simulink model "hcu_main_ADASwEPS"  (Simulink 8.2)
settings: Solver=FixedStepDiscrete  StartTime=0.0  StopTime=inf  FixedStep=0.001  RelTol=1e-3
PostLoadFcn:
  | , if any(exist('dsrtsu_mdlpostloadfcn', 'file') == [2, 3, 6]), try dsrtsu_mdlpostloadfcn('Execute', bdroot); catch fprintf('Error in PostLoadFcn (dsrtsu_mdlpostloadfcn) for model "%s":\n %s\n', bdroot, lasterr); end, end,
values from neighbouring files (symbols this model uses):
  C_TASK_1MS_S = (	C_TICK_TIME_S       )    [hcu_local_hdr.m]    (also in temp_ovrd_values.m = double(	0.001                  ))
  C_TASK_5MS_S = (	C_TICK_TIME_S      	)    [hcu_local_hdr.m]
  ENUM_ADASLFCSTATUS_OFF = uint8(  0  )    [hcu_local_hdr.m]
  ENUM_ADASLFCSTATUS_STANDBY = uint8(  1  )    [hcu_local_hdr.m]
  ENUM_ADASLKASTATUS_ACTIVE = uint8(  2  )    [hcu_local_hdr.m]
  ENUM_ADASLKASTATUS_OFF = uint8(  0  )    [hcu_local_hdr.m]
  ENUM_ADASLKASTATUS_STANDBY = uint8(  1  )    [hcu_local_hdr.m]
  ENUM_EPSMODEREQ_ANGLE = uint8(  1  )    [hcu_local_hdr.m]
  ENUM_EPSMODEREQ_INTERNAL = uint8(  0  )    [hcu_local_hdr.m]
  ENUM_EPSMODEREQ_TORQUE = uint8(  2  )    [hcu_local_hdr.m]
  ENUM_GEARPOSN_1ST = uint8(  1  )    [hcu_local_hdr.m]
  ENUM_GEARPOSN_2ND = uint8(  2  )    [hcu_local_hdr.m]
  ENUM_GEARPOSN_3RD = uint8(  3  )    [hcu_local_hdr.m]
  ENUM_GEARPOSN_4TH = uint8(  4  )    [hcu_local_hdr.m]
  ENUM_GEARPOSN_5TH = uint8(  5  )    [hcu_local_hdr.m]
  ENUM_GEARPOSN_6TH = uint8(  6  )    [hcu_local_hdr.m]
  ENUM_GEARPOSN_PN = uint8(  0  )    [hcu_local_hdr.m]
  ENUM_GEARPOSN_R = uint8(  7  )    [hcu_local_hdr.m]
  FALSE = boolean( 0 )    [hcu_local_hdr.m]
  TRUE = boolean( 1 )    [hcu_local_hdr.m]
undefined symbols (not defined in the file or in its folder): AACC_DistCtrlIMult_X_mps2, AACC_DistCtrlPMult_X_mps2, AACC_GearActual_enum, AACC_SpdCtrlIMult_X_mps2, AACC_SpdCtrlPMult_X_mps2, AACC_VehSpd_kph, AISP_EPSCurrent_pct, AISP_TqASensorDelta_pct, AISP_TqBSensorDelta_pct, ENUM_ACCSTATUS_ACTIVE, ENUM_ACCSTATUS_OFF, ENUM_ACCSTATUS_STANDBY, ENUM_ADASLFCSTATUS_ACTIVE, ENUM_ADASLFCSTATUS_TRANSITION, ENUM_LFCCCONTSTATUS_ACTIVE, ENUM_LFCCCONTSTATUS_NOTAVAIL_TEMP, ENUM_LFCCCONTSTATUS_OFF, ENUM_LFCCCONTSTATUS_READY, ENUM_LFCCCONTSTATUS_TRANSITION, ENUM_LKACCONTSTATUS_ACTIVE, ENUM_LKACCONTSTATUS_NOTAVAIL_TEMP, ENUM_LKACCONTSTATUS_OFF, ENUM_LKACCONTSTATUS_READY, KACC_AcclReqMax_g, KACC_AcclReqMin_g, KACC_ACCSetTimeGapDef1_s, KACC_ACCSetTimeGapDef2_s, KACC_ACCSetTimeGapDef3_s, KACC_ACCSetTimeGapDef4_s, KACC_ACCSetTimeGapDef5_s, KACC_AirDensity_kgpm3, KACC_AirDragCoef_rat, KACC_CommandsOn_flg, KACC_CruzSpdChgTimeThres_s, KACC_DecReqSwOffThres_Nm, KACC_DecReqSwOnThres_Nm, KACC_DistCtrlAdjTime_s, KACC_DistCtrlCalRate_s, KACC_DistCtrlIC_mps2, KACC_DistCtrlIGain_rat, KACC_DistCtrlIMax_mps2, KACC_DistCtrlIMin_mps2, KACC_DistCtrlIRest_flg, KACC_DistCtrlKGain_rat, KACC_DistCtrlPause_flg, KACC_DistCtrlPGain_rat, KACC_FinalDriveEff_pct, KACC_FinalDriveRatio_rat, KACC_FrontalArea_m2, KACC_GearBoxEff_pct, KACC_LongPushSpdChg_kph, KACC_MaxAccSetSpd_kph, KACC_MinAccSetSpd_kph, KACC_SetAllowSpdLim_kph, KACC_SpdCtrlAdjTime_s, KACC_SpdCtrlCalRate_s, KACC_SpdCtrlIC_mps2, KACC_SpdCtrlIGain_rat, KACC_SpdCtrlIMax_mps2, KACC_SpdCtrlIMin_mps2 ... (+26)
libraries: simulink x54, adas_lib x6, rti1401lib_dio_type3 x4, rtimmsu_dsrtlib x3, hcu_lib x2, aeb x1, ddm x1, dfr x1, dgi x1, dhp x1, dinr x1, dip x1
(part 1 of 9)
settings Model: DSRTSU_INTERNAL_RTI_VER=460  DSRTSU_INTERNAL_RTI_TYPE=rti1401  RTICANMMDATA=struct('GeneralSetupData',struct('modelroot','D:\HAITEC\SVN\trunk\ADAS_Softwares\HTDragon\software\sw_development\arch','generalsettings',struct('filesettings',struct('destfolder',struct('Name','..\build\RTICANMM_FILES_ADASwEPS','Check',1),'buildfolder',struct('Name','.','Check',1),'AbsDestfolder',struct('Name','D:\HAITEC\SVN\trunk\ADAS_Softwares\HTDragon\software\sw_development\build\RTICANMM_FILES_ADASwEPS'),'AbsBuildfolder',struct('Name','D:\HAITEC\SVN\trunk\ADAS_Softwares\HTDragon\software\sw_development\arch'))),'options',struct('addpaths',1,'rmpaths',1,'addtrcexclusion',1,'cannavigator',struct('checkmonitoring',1),'show_usrtrc',0,'use_usrtrc',0,'addpath2usrmk',1),'advanced',struct('options',[1 1 1 1 1 1 1 1 1 1 1 1 1 1 1 1 1 1 1 1 1 1 1 1 1 1 1 1 1 1 1 1 1 1 1 1 1 1 1 1 1 1 1 1 1 1 1 1 1 1 1 1 1 1 1 1 1 1 1 1 1 1 1 1 1 1 1 1 1 1 1 1 1 1 1 1 1 1 1 1 1 1 1 1 1 1 1 1 1 1 1 1 1 1 1 1 1 1 1 1]),'MPSetup',{{}},'modelname','hcu_main_ADASwEPS','blockdata',struct('generalsettings',struct('filesettings',struct('destfolder',struct('Name','.','Check',1),'AbsDestfolder',struct('Name','T:\TOOL_SOURCES\CANnedy\m'),'buildfolder',struct('Name','.','Check',1),'AbsBuildfolder',struct('Name','C:\MATLAB6p5\work'))),'options',struct('addpaths',1,'rmpaths',1,'addpath2usrmk',1),'modelname','rticanmmlib','modelroot','T:\TOOL_SOURCES\CANnedy\m'),'MMType','RTICANMM','block',['hcu_main_ADASwEPS/RTICANMM' char(10) 'GeneralSetup'],'userdata',struct('HostServiceChannelID',{{'CAN_2',[],'CAN_1'}}),'RTI',struct('Type','RTI1401','Ver','7.4','Date','02-May-2015'),'version','4.1.736021.4900694444'))  DSRTSU_INTERNAL_RTIFPGA=50  Creator=11116  LastModifiedBy=14014  BufferReuse=off
settings DataIOCC: SignalLoggingSaveFormat=Dataset  SaveOutput=off  SaveTime=off
settings OptimizationCC: BlockReduction=off  OptimizeBlockIOStorage=off  BufferReuse=off  ExpressionFolding=off  ExpressionDepthLimit=128  LocalBlockOutputs=off
settings DebuggingCC: ParameterPrecisionLossMsg=none  FcnCallInpInsideContextMsg=EnableAllAsError  StateNameClashWarn=none
settings HardwareCC: ProdIntDivRoundTo=Zero  ProdEndianess=BigEndian  ProdHWDeviceType=Generic->Custom  TargetIntDivRoundTo=Zero  TargetEndianess=BigEndian  TargetHWDeviceType=Generic->Custom
settings RTWCC: SystemTargetFile=rti1401.tlc  MakeCommand=make_rti  TemplateMakefile=rti1401.tmf  Description=dSPACE DS1401 Hardware Platform  ProcessScript=rti1401_make_rtw_hook
settings STFCustomTargetCC: CodeReplacementLibrary=ANSI_C  ParMdlRefBuildCompliant=on  GeneratePreprocessorConditionals=Disable all  SystemTargetFile=rti1401.tlc
settings GRTTargetCC: CompOptLevelCompliant=off  ConcurrentExecutionCompliant=off  MatFileLogging=off  ExtModeMexFile=noextcomm
settings CustomProperty: DataType=RTWOptions_EnumType_C__Program Files_dSPACE RCPHIL 2015-A_MATLAB_RTI_RTI1401_TLC_rti1401_1InitialSimState  Value=RUN
settings EnumStrPairs: String=RUN

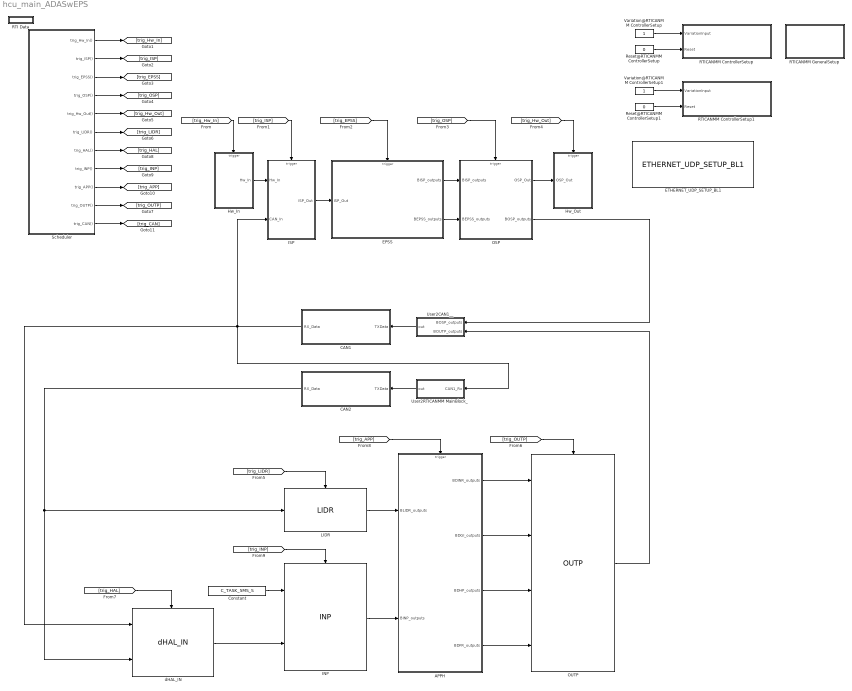
== system hcu_main_ADASwEPS ==
  APPH : Subsystem
      settings: RTWSystemCode=Nonreusable function  RTWFcnNameOpts=Use subsystem name  RTWFileNameOpts=Use subsystem name
  CAN1 : Subsystem  InitFcn=rticanmm_blockfcn('InitFcn', 'CANnedy', gcb)  ClipboardFcn=rticanmm_blockfcn('ClipboardFcn', 'CANnedy', gcb)  mask(RTICANMM){DSProperties=struct('RTI',struct('Version',uint32(1),'BlockType',struct('isSLSource',uint8(1),'isSLSink',uint8(1),'isHWSource',uint8(0),'isHWSink',uint8(0),'isSetup',uint8(0),'isInline',uint8(1),'isNonInline',uint8(0),'isInterrupt',uint8(0),'isChannelwise',uint8(0)),'IOBoardType','RTICANMM','UnitType','RTICANMM','Identifier','Mainblock','DialogType','SL','BlockSet','RTICANMM','SlaveProcessor','CAN')), CANMMProperties=struct('RTICANMMVersion','4.1','RTICANMMVersionIntern','4.1.736021.4900694444','RTICANMMDate','02-May-2015','Settings','RTICANMM_MAIN_CAN_1','UserTracePath','','ModelPath','D:\HAITEC\SVN\trunk\ADAS_Softwares\HTDragon\software\sw_development\arch','filesettings',struct('FileName','..\..\..\..\CAN\ADAS_CAN1_Mule1_BSGEMS_MVCU_MEPS_20160121_db.dbc','IsRelative',1,'ClusterId',1,'ClusterList',{{'default'}},'destfolder',struct('Name','..\build\RTICANMM_FILES_ADASwEPS','Check',1),'buildfolder',struct('Name','.','Check',1),'onlyfreerawcapture',0,'overlapping2variant',0,'canfdsupport',0,'shortestJ2container',1),'onlyfreerawcapture',0,'Board',['CAN Type 1'],'BoardNum','1','ChannelNum','1','Variation','1','SetupId','CAN_1','MARK',['87FB4930AEF4A7AAC589F26C78E4F4';'72FEF8353FB46D1087126C7939F170';'8EAD2A2CD2FE1AE61023D4FA11BE9C';'5611A927C2EC9CAF50988DCF8D639B';'13F55C241594A2B2B8AC667E2018BB'],'date','23-Jan-2016','clock',['23.01.2016 09:32:58'],'recreate',0,'RTIVER','RTI1401','j1939',0,'TRC',struct('include',1),'rtsupport',struct('XMLFile','D:\HAITEC\SVN\trunk\ADAS_Softwares\HTDragon\software\sw_development\build\RTICANMM_FILES_ADASwEPS\RTICANMM_MAIN_CAN_1.xml','DBCXML',struct('Path','D:\HAITEC\SVN\trunk\ADAS_Softwares\HTDragon\software\sw_development\build\RTICANMM_FILES_ADASwEPS\RTICANMM_MAIN_CAN_1_dbc.xml','support',1,'Name','ADAS_CAN1_Mule1_BSGEMS_MVCU_MEPS_20160121_db.dbc','Date',['22-一月-2016 09:11:58'],'Type','standard','DBCSupport','ON'))), CANMMType=CANnedy, CANMMUserTraceMerged=off, CANMMUserTracePath=, CANMMChannelNum=1, CANMMBoardNum=1, CANMMDestFolder=..\build\RTICANMM_FILES_ADASwEPS, CANMMFolder=., CANMMSetupId=CAN_1, CANMMsave2mat=['87FB4930AEF4A7AAC589F26C78E4F4';'72FEF8353FB46D1087126C7939F170';'8EAD2A2CD2FE1AE61023D4FA11BE9C';'5611A927C2EC9CAF50988DCF8D639B';'13F55C241594A2B2B8AC667E2018BB'], CANMMName=CAN_1, CANMMSettings=RTICANMM_MAIN_CAN_1, CANMMIntermediateTag=RTICANMM_MAIN_CAN_1_intermediate, CANMMsfcnname=RTICANMM_MAIN_CAN_1}
      mask init:
      | rticanmm_initfcn(gcb, CANMMType, CANMMsfcnname)
      settings: AttributesFormatString=CAN_1[CAN_1]: DS1401_B1_C1_V1  CopyFcn=rticanmm_blockfcn('CopyFcn', 'CANnedy', gcb)  DeleteFcn=rticanmm_blockfcn('DeleteFcn', 'CANnedy', gcb)  ModelCloseFcn=rticanmm_blockfcn('ModelCloseFcn', 'CANnedy', gcb)  NameChangeFcn=rticanmm_blockfcn('NameChangeFcn', 'CANnedy', gcb)  OpenFcn=try, rticanmm_main_gui('create',gcb); ; catch,errordlg({lasterr, '','Please check your RTI installation.'},['Error: ' upper(bdroot)], 'replace'); end  MoveFcn=rticanmm_blockfcn('MoveFcn', 'CANnedy', gcb)
      mask Help: eval('rticanmm_quickstart(''create'', gcb);', 'disp(lasterr);')
      mask Display:
      | disp(sprintf('RTI CAN\nMultiMessage\nMainSetup'))
      | port_label('input', 1, 'TX Data')
      | port_label('output', 1, 'RX Data')
  CAN2 : Subsystem  InitFcn=rticanmm_blockfcn('InitFcn', 'CANnedy', gcb)  ClipboardFcn=rticanmm_blockfcn('ClipboardFcn', 'CANnedy', gcb)  mask(RTICANMM){DSProperties=struct('RTI',struct('Version',uint32(1),'BlockType',struct('isSLSource',uint8(1),'isSLSink',uint8(1),'isHWSource',uint8(0),'isHWSink',uint8(0),'isSetup',uint8(0),'isInline',uint8(1),'isNonInline',uint8(0),'isInterrupt',uint8(0),'isChannelwise',uint8(0)),'IOBoardType','RTICANMM','UnitType','RTICANMM','Identifier','Mainblock','DialogType','SL','BlockSet','RTICANMM','SlaveProcessor','CAN')), CANMMProperties=struct('RTICANMMVersion','4.1','RTICANMMVersionIntern','4.1.736021.4900694444','RTICANMMDate','02-May-2015','Settings','RTICANMM_MAIN_CAN_2','UserTracePath','','ModelPath','D:\HAITEC\SVN\trunk\ADAS_Softwares\HTDragon\software\sw_development\arch','filesettings',struct('FileName','..\..\..\..\CAN\IDIADA_CAN2_Chimo.dbc','IsRelative',1,'ClusterId',1,'ClusterList',{{'default'}},'destfolder',struct('Name','..\build\RTICANMM_FILES_ADASwEPS','Check',1),'buildfolder',struct('Name','.','Check',1),'onlyfreerawcapture',0,'overlapping2variant',0,'canfdsupport',0,'shortestJ2container',1),'onlyfreerawcapture',0,'Board',['CAN Type 1'],'BoardNum','1','ChannelNum','2','Variation','1','SetupId','CAN_2','MARK',['4E53C812CB570F3DF79E35A61EC1B4';'A1237348498B5F46CB73D5EF117ED2';'77465375665041D5559DC8396B874D';'03CE9519A3063C2C69A49AF64F1FBA';'05E25404A442834EF54FA0177E6CB6'],'date','23-Jan-2016','clock',['23.01.2016 09:38:04'],'recreate',0,'RTIVER','RTI1401','j1939',0,'TRC',struct('include',1),'rtsupport',struct('XMLFile','D:\HAITEC\SVN\trunk\ADAS_Softwares\HTDragon\software\sw_development\build\RTICANMM_FILES_ADASwEPS\RTICANMM_MAIN_CAN_2.xml','DBCXML',struct('Path','D:\HAITEC\SVN\trunk\ADAS_Softwares\HTDragon\software\sw_development\build\RTICANMM_FILES_ADASwEPS\RTICANMM_MAIN_CAN_2_dbc.xml','support',1,'Name','IDIADA_CAN2_Chimo.dbc','Date',['23-一月-2016 09:07:49'],'Type','standard','DBCSupport','ON'))), CANMMType=CANnedy, CANMMUserTraceMerged=off, CANMMUserTracePath=, CANMMChannelNum=2, CANMMBoardNum=1, CANMMDestFolder=..\build\RTICANMM_FILES_ADASwEPS, CANMMFolder=., CANMMSetupId=CAN_2, CANMMsave2mat=['4E53C812CB570F3DF79E35A61EC1B4';'A1237348498B5F46CB73D5EF117ED2';'77465375665041D5559DC8396B874D';'03CE9519A3063C2C69A49AF64F1FBA';'05E25404A442834EF54FA0177E6CB6'], CANMMName=CAN_2, CANMMSettings=RTICANMM_MAIN_CAN_2, CANMMIntermediateTag=RTICANMM_MAIN_CAN_2_intermediate, CANMMsfcnname=RTICANMM_MAIN_CAN_2}
      mask init:
      | rticanmm_initfcn(gcb, CANMMType, CANMMsfcnname)
      settings: AttributesFormatString=CAN_2[CAN_2]: DS1401_B1_C2_V1  CopyFcn=rticanmm_blockfcn('CopyFcn', 'CANnedy', gcb)  DeleteFcn=rticanmm_blockfcn('DeleteFcn', 'CANnedy', gcb)  ModelCloseFcn=rticanmm_blockfcn('ModelCloseFcn', 'CANnedy', gcb)  NameChangeFcn=rticanmm_blockfcn('NameChangeFcn', 'CANnedy', gcb)  OpenFcn=try, rticanmm_main_gui('create',gcb); ; catch,errordlg({lasterr, '','Please check your RTI installation.'},['Error: ' upper(bdroot)], 'replace'); end  MoveFcn=rticanmm_blockfcn('MoveFcn', 'CANnedy', gcb)
      mask Help: eval('rticanmm_quickstart(''create'', gcb);', 'disp(lasterr);')
      mask Display:
      | disp(sprintf('RTI CAN\nMultiMessage\nMainSetup'))
      | port_label('input', 1, 'TX Data')
      | port_label('output', 1, 'RX Data')
  Constant : Constant  Value=C_TASK_5MS_S
  EPSS : Subsystem
      settings: RTWSystemCode=Nonreusable function  RTWFcnNameOpts=Use subsystem name  RTWFileNameOpts=Use subsystem name
  ETHERNET_UDP_SETUP_BL1 : rtiethernetudplib/ETHERNET_UDP_SETUP_BL1  DSProperties=struct('RTI',struct('Version',uint32(1),'BlockType',struct('isSLSource',uint8(0),'isSLSink',uint8(0),'isHWSource',uint8(0),'isHWSink',uint8(0),'isSetup',uint8(0),'isInline',uint8(1),'isNonInline',uint8(1),'isInterrupt',uint8(0),'isChannelwise',uint8(0)),'IOBoardType','DSETHERNETUDP','UnitType','ETHUDP','Identifier','SETUP','DialogType','ML','BlockSet','RTIETHERNETUDP','SlaveProcessor','NONE'))  RTIBlockInterface=struct('OutputPortsActive',0,'OutputPortsWidth',int32(1),'DialogFcn','rtiethernetudpsetupgui','InitLevel',3,'BlockDisplay',{{['Ethernet UDP Setup\nInterface Name: rti_ethernet_interface_name\nBoard Type: ETH Type 1\nModule: 1\nLocal IP Address: 192.168.140.11'],'center'}},'IconTransparency','on','BlockName',struct('Token',{{'ETHERNET_UDP_SETUP_BL1'}}))  RTIBlockParameters=struct('BoardType',{{1,'OFF',[]}},'ModuleNo',{{1,'ON',[1 16]}},'ChannelNo',{{1,'ON',[1 2]}},'InterfaceName',{{'rti_ethernet_interface_name','OFF',[]}},'LocalIpAddress',{{'192.168.140.11','OFF',[]}},'EnableSocket1',{{1,'OFF',[0 1]}},'LocalPortSocket1',{{'30000','OFF',[0 65535]}},'RemoteIpAddrSocket1',{{'192.168.140.10','OFF',[]}},'RemotePortSocket1',{{'30000','OFF',[0 65535]}},'EnableSocket2',{{1,'OFF',[0 1]}},'LocalPortSocket2',{{'30000','OFF',[0 65535]}},'RemoteIpAddrSocket2',{{'0.0.0.0','OFF',[]}},'RemotePortSocket2',{{'0','OFF',[0 65535]}},'EnableSocket3',{{0,'OFF',[0 1]}},'LocalPortSocket3',{{'5002','OFF',[0 65535]}},'RemoteIpAddrSocket3',{{'XXX.XXX.XXX.XXX','OFF',[]}},'RemotePortSocket3',{{'5002','OFF',[0 65535]}},'EnableSocket4',{{0,'OFF',[0 1]}},'LocalPortSocket4',{{'5003','OFF',[0 65535]}},'RemoteIpAddrSocket4',{{'XXX.XXX.XXX.XXX','OFF',[]}},'RemotePortSocket4',{{'5003','OFF',[0 65535]}},'LocalIpAddrHex',{{3232271371,'OFF',[]}},'RemoteIpAddrSocket1Hex',{{3232271370,'OFF',[]}},'RemoteIpAddrSocket2Hex',{{0,'OFF',[]}},'RemoteIpAddrSocket3Hex',{{0,'OFF',[]}},'RemoteIpAddrSocket4Hex',{{0,'OFF',[]}})  RTISFcnParameters=struct('BoardType','double','ModuleNo','double','ChannelNo','double','InterfaceName','char','LocalIpAddress','char','EnableSocket1','double','LocalPortSocket1','double','RemoteIpAddrSocket1','char','RemotePortSocket1','double','EnableSocket2','double','LocalPortSocket2','double','RemoteIpAddrSocket2','char','RemotePortSocket2','double','EnableSocket3','double','LocalPortSocket3','double','RemoteIpAddrSocket3','char','RemotePortSocket3','double','EnableSocket4','double','LocalPortSocket4','double','RemoteIpAddrSocket4','char','RemotePortSocket4','double','LocalIpAddrHex','double','RemoteIpAddrSocket1Hex','double','RemoteIpAddrSocket2Hex','double','RemoteIpAddrSocket3Hex','double','RemoteIpAddrSocket4Hex','double')  RTIBlockParaDefault=struct('BoardType',1,'ModuleNo',1,'ChannelNo',1,'InterfaceName','rti_ethernet_interface_name','LocalIpAddress','XXX.XXX.XXX.XXX','EnableSocket1',0,'LocalPortSocket1',5000,'RemoteIpAddrSocket1','XXX.XXX.XXX.XXX','RemotePortSocket1',5000,'EnableSocket2',0,'LocalPortSocket2',5001,'RemoteIpAddrSocket2','XXX.XXX.XXX.XXX','RemotePortSocket2',5001,'EnableSocket3',0,'LocalPortSocket3',5002,'RemoteIpAddrSocket3','XXX.XXX.XXX.XXX','RemotePortSocket3',5002,'EnableSocket4',0,'LocalPortSocket4',5003,'RemoteIpAddrSocket4','XXX.XXX.XXX.XXX','RemotePortSocket4',5003,'LocalIpAddrHex',0,'RemoteIpAddrSocket1Hex',0,'RemoteIpAddrSocket2Hex',0,'RemoteIpAddrSocket3Hex',0,'RemoteIpAddrSocket4Hex',0)
  Hw_In : Subsystem
  Hw_Out : Subsystem
  INP : inp/INP
  ISP : Subsystem
  LIDR : lidr/LIDR
  OSP : Subsystem
  OUTP : outp/OUTP
  RTI Data : Subsystem  Tag=struct('RTIDataServer',struct('RTIDataServerVs','2','RTIModelDescription','struct(''main'',''hcu_main_ADASwEPS'',''sub'','''',''isMp'',0)'))  LoadFcn="if exist('rtidc'), try,  rtidc('DataHostBlockClbLoad', gcbh); catch, disp(['Warning: ''LoadFcn'' for RTI Data block failed: ' lasterr]); end, end,"  mask(RTI_DATA_HOST){}
      mask help:
      | RTI Data Block.
      | This block is used by RTI to store internal model-dependent data.
      | Please keep this block on the root level of the model. Deleting this block will result in data loss.
      |
      | NEVER DELETE OR COPY THIS BLOCK!
      settings: CopyFcn="if exist('rtidc'), try,  rtidc('DataHostBlockClbCopy', gcbh); catch, disp(['Warning: ''CopyFcn'' for RTI Data block failed: ' lasterr]); end, end,"  DeleteFcn="if exist('rtidc'), try,  rtidc('DataHostBlockClbDelete', gcbh); catch, disp(['Warning: ''DeleteFcn'' for RTI Data block failed: ' lasterr]); end, end,"  ModelCloseFcn="if exist('rtidc'), try,  rtidc('DataHostBlockClbModelClose', gcbh); catch, disp(['Warning: ''ModelCloseFcn'' for RTI Data block failed: ' lasterr]); end, end,"  PreSaveFcn="if exist('rtidc'), try,  rtidc('DataHostBlockClbPreSave', gcbh); catch, disp(['Warning: ''PreSaveFcn'' for RTI Data block failed: ' lasterr]); end, end,"  PostSaveFcn="if exist('rtidc'), try,  rtidc('DataHostBlockClbPostSave', gcbh); catch, disp(['Warning: ''PostSaveFcn'' for RTI Data block failed: ' lasterr]); end, end,"  NameChangeFcn="if exist('rtidc'), try,  rtidc('DataHostBlockClbNameChange', gcbh); catch, disp(['Warning: ''NameChangeFcn'' for RTI Data block failed: ' lasterr]); end, end,"
      mask Help:
      | RTI Data Block.
      | This block is used by RTI to store internal model-dependent data.
      | Please keep this block on the root level of the model. Deleting this block will result in data loss.
      | 
      | NEVER DELETE OR COPY THIS BLOCK!
      mask Display:
      | text(0.5, 0.5, 'RTI Data', 'HorizontalAlignment', 'center');
      | plot([1 0]);
  RTICANMM ControllerSetup : Subsystem  InitFcn=rticanmm_blockfcn('InitFcn', 'CANnedySetup', gcb)  ClipboardFcn=rticanmm_blockfcn('ClipboardFcn', 'CANnedySetup', gcb)  mask(RTICANMM){DSProperties=struct('RTI',struct('Version',uint32(1),'BlockType',struct('isSLSource',uint8(1),'isSLSink',uint8(1),'isHWSource',uint8(0),'isHWSink',uint8(0),'isSetup',uint8(0),'isInline',uint8(1),'isNonInline',uint8(0),'isInterrupt',uint8(0),'isChannelwise',uint8(0)),'IOBoardType','RTICANMM','UnitType','RTICANMM','Identifier','BUSSETUP','DialogType','SL','BlockSet','RTICANMM','SlaveProcessor','CAN')), CANMMProperties=struct('cannedy',struct('data',struct('options',struct('controllername','CAN_1','controllernameautomatic',[],'loglevel','0','checkrealtime',0,'checkchangebaudrate',0,'sampletime','1.000','CANControllerStatus',0,'NumberofStuffErr',0,'NumberofFormErr',0,'NumberofAckErr',0,'NumberofBit0Err',0,'NumberofsuccrecRX',0,'Numberofsuccsent',0,'NumberofBit1Err',0,'NumberofCRCErr',0,'NumberoflostRX',0,'Busoff',0,'Busload',0,'OperationPending',0,'TxRetryCount',3,'addtrcexclusion',logical(1),'cannavigator',struct('checkmonitoring',0,'checkinternmonitoring',0),'show_usrtrc',0,'use_usrtrc',0,'checkchangebaudrateFD',0,'errorframegeneration',0,'efgenabled',0),'modelroot','D:\ADAS\ADAS\trunk\Demo\AI\ACM_d2','generalsettings',struct('setupdata',struct('board',['CAN Type 1'],'boardno',1,'channelno',1,'Type','STD','transceiver','ISO11898-2','busconfig','0x0','feedthrough','false','resistance',struct('r120',0,'roff',1,'r16',1,'r10',0),'baudrate','500','Frequency',[24 36],'samplemode',1,'commChannelTJA1041',6,'config',struct('standard',1,'advanced',0,'register',struct('btr0','0xC0','btr1','0x6F','sp','70','sjw','3','tseg1','15','tseg2','6','brp','0','smpl','0','btr0_36','0x41','btr1_36','0x1E','sp_36','88','sjw_36','1','tseg1_36','14','tseg2_36','1','brp_36','1','smpl_36','0','btr0_64','0x43','btr1_64','0x1C','sp_64','87','sjw_64','1','tseg1_64','12','tseg2_64','1','brp_64','3','smpl_64','0')),'channelcfg',struct('INTENDISABLE','CAN_INT_DISABLE','intenable',0),'SETUPID','RTICANMM_CAN_1_ID','CONTROLLER_ID','CANMM_CTL_SETUP_CAN_1','mainblock_includefile','RTICANMM_SETUP_CAN_1','canfdenable',0,'canfdboardselected',0,'slotno',1,'moduletype','DS4342','baudrateFD','4000','termination','TERMINATION_OFF'),'filesettings',struct('destfolder',struct('Name','RTICANMM_FILES','Check',1),'buildfolder',struct('Name','.','Check',1))),'advanced',struct('options',[1 1 1 1 1 1 1 1 1 1 1 1 1 1 1 1 1 1 1 1 1 1 1 1 1 1 1 1 1 1 1 1 1 1 1 1 1 1 1 1 1 1 1 1 1 1 1 1 1 1 1 1 1 1 1 1 1 1 1 1 1 1 1 1 1 1 1 1 1 1 1 1 1 1 1 1 1 1 1 1 1 1 1 1 1 1 1 1 1 1 1 1 1 1 1 1 1 1 1 1]),'partialnetdata',struct('switchedon',0,'format','STD','idmask',['XXXXX XXXXXXXX XXXXXXXX XXXXXXXX'],'idcode','0','idfilter','0','datamaskused',0,'datalength','0','datamask','0x0000000000000000','partialnetworkenable',0)),'blk',['hcu_main_ADASwEPS/RTICANMM' char(10) 'ControllerSetup'],'allgeneratedfiles',{{'D:\HAITEC\SVN\trunk\ADAS_Softwares\HTDragon\software\sw_development\build\RTICANMM_FILES_ADASwEPS\RTICANMM_SETUP_CAN_1.c','D:\HAITEC\SVN\trunk\ADAS_Softwares\HTDragon\software\sw_development\build\RTICANMM_FILES_ADASwEPS\RTICANMM_SETUP_CAN_1.h','d:\haitec\svn\trunk\adas_softwares\htdragon\software\sw_development\build\rticanmm_files_adasweps\rticanmm_setup_can_1.mexw32'}},'ismp',logical(0),'BlockDataVersion','0.8.0','recreate',0),'CANnedynew',0,'CANnedySettings','CAN_1','GeneratedFiles',{{'D:\HAITEC\SVN\trunk\ADAS_Softwares\HTDragon\software\sw_development\build\RTICANMM_FILES_ADASwEPS\RTICANMM_SETUP_CAN_1.c','D:\HAITEC\SVN\trunk\ADAS_Softwares\HTDragon\software\sw_development\build\RTICANMM_FILES_ADASwEPS\RTICANMM_SETUP_CAN_1.h','d:\haitec\svn\trunk\adas_softwares\htdragon\software\sw_development\build\rticanmm_files_adasweps\rticanmm_setup_can_1.mexw32'}},'SFCN','RTICANMM_SETUP_CAN_1.c','HostService',struct('Tags',struct('DATA','RTICANMM_MonitorData','TimeStampGlobal','RTICANMM_MonitoringTimeStamp','TimeStampGlobalEnable','RTICANMM_MonitoringTimeStampEnable','Enable','CANMMMonitor_CAN_1','TimeStamp','MonitoringTimeStamp_CAN_1'),'DATA',struct('Length',18),'Info',struct('Desc',{'ID','Service','Data1','Data2','Data3','Data4','Data5','Data6','Data7','Data8','Data9','Data10','Data11','Data12','Data13','Data14','Data15','Data16'}),'Names',struct('TimeStampGlobal','TimeStamp','TimeStampGlobalEnable','TimeStamp_Enable','Enable','Monitoring_Enable','TimeStamp','Monitoring_TimeStamp'),'ChannelID',3)), CANMMType=CANnedySetup, CANMMFolder=D:\HAITEC\SVN\trunk\ADAS_Softwares\HTDragon\software\sw_development\arch, CANMMDestFolder=..\build\RTICANMM_FILES_ADASwEPS, CANMMSettings=CAN_1, CANMMSFcn=RTICANMM_SETUP_CAN_1, CANMMBoard=DS1401, CANMMBoardNum=1, CANMMChannel=1}
      settings: AttributesFormatString=%<CANMMSettings>: %<CANMMBoard>_B%<CANMMBoardNum>_C%<CANMMChannel>  CopyFcn=rticanmm_blockfcn('CopyFcn', 'CANnedySetup', gcb)  DeleteFcn=rticanmm_blockfcn('DeleteFcn', 'CANnedySetup', gcb)  ModelCloseFcn=rticanmm_blockfcn('ModelCloseFcn', 'CANnedySetup', gcb)  NameChangeFcn=rticanmm_blockfcn('NameChangeFcn', 'CANnedySetup', gcb)  OpenFcn=try, rticanmm_setup_gui('create',gcb); ; catch,errordlg({lasterr, '','Please check your RTI installation.'},['Error: ' upper(bdroot)], 'replace'); end  MoveFcn=rticanmm_blockfcn('MoveFcn', 'CANnedySetup', gcb)
      mask Help: eval('rticanmm_quickstart(''create'', gcb);', 'disp(lasterr);')
      mask Display:
      | disp('RTI CAN\nMultiMessage\nControllerSetup')
      | 
      | port_label('input', 1 , 'Variation')
      | port_label('input', 2 , 'Reset')
  RTICANMM ControllerSetup1 : Subsystem  InitFcn=rticanmm_blockfcn('InitFcn', 'CANnedySetup', gcb)  ClipboardFcn=rticanmm_blockfcn('ClipboardFcn', 'CANnedySetup', gcb)  mask(RTICANMM){DSProperties=struct('RTI',struct('Version',uint32(1),'BlockType',struct('isSLSource',uint8(1),'isSLSink',uint8(1),'isHWSource',uint8(0),'isHWSink',uint8(0),'isSetup',uint8(0),'isInline',uint8(1),'isNonInline',uint8(0),'isInterrupt',uint8(0),'isChannelwise',uint8(0)),'IOBoardType','RTICANMM','UnitType','RTICANMM','Identifier','BUSSETUP','DialogType','SL','BlockSet','RTICANMM','SlaveProcessor','CAN')), CANMMProperties=struct('cannedy',struct('data',struct('options',struct('controllername','CAN_2','controllernameautomatic',[],'loglevel','0','checkrealtime',0,'checkchangebaudrate',0,'sampletime','1.000','CANControllerStatus',0,'NumberofStuffErr',0,'NumberofFormErr',0,'NumberofAckErr',0,'NumberofBit0Err',0,'NumberofsuccrecRX',0,'Numberofsuccsent',0,'NumberofBit1Err',0,'NumberofCRCErr',0,'NumberoflostRX',0,'Busoff',0,'Busload',0,'OperationPending',0,'TxRetryCount',3,'addtrcexclusion',logical(1),'cannavigator',struct('checkmonitoring',0,'checkinternmonitoring',0),'show_usrtrc',0,'use_usrtrc',0,'checkchangebaudrateFD',0,'errorframegeneration',0,'efgenabled',0),'modelroot','D:\ActiveSafetyDepartment\SVN\trunk\Demo\AI\ACM_d5','generalsettings',struct('setupdata',struct('board',['CAN Type 1'],'boardno',1,'channelno',2,'Type','STD','transceiver','ISO11898-2','busconfig','0x0','feedthrough','false','resistance',struct('r120',0,'roff',1,'r16',1,'r10',0),'baudrate','500','Frequency',[24 36],'samplemode',1,'commChannelTJA1041',6,'config',struct('standard',1,'advanced',0,'register',struct('btr0','0xC0','btr1','0x6F','sp','70','sjw','3','tseg1','15','tseg2','6','brp','0','smpl','0','btr0_36','0x41','btr1_36','0x1E','sp_36','88','sjw_36','1','tseg1_36','14','tseg2_36','1','brp_36','1','smpl_36','0','btr0_64','0x43','btr1_64','0x1C','sp_64','87','sjw_64','1','tseg1_64','12','tseg2_64','1','brp_64','3','smpl_64','0')),'channelcfg',struct('INTENDISABLE','CAN_INT_DISABLE','intenable',0),'SETUPID','RTICANMM_CAN_2_ID','CONTROLLER_ID','CANMM_CTL_SETUP_CAN_2','mainblock_includefile','RTICANMM_SETUP_CAN_2','canfdenable',0,'canfdboardselected',0,'slotno',1,'moduletype','DS4342','baudrateFD','4000','termination','TERMINATION_OFF'),'filesettings',struct('destfolder',struct('Name','RTICANMM_FILES','Check',1),'buildfolder',struct('Name','.','Check',1))),'advanced',struct('options',[1 1 1 1 1 1 1 1 1 1 1 1 1 1 1 1 1 1 1 1 1 1 1 1 1 1 1 1 1 1 1 1 1 1 1 1 1 1 1 1 1 1 1 1 1 1 1 1 1 1 1 1 1 1 1 1 1 1 1 1 1 1 1 1 1 1 1 1 1 1 1 1 1 1 1 1 1 1 1 1 1 1 1 1 1 1 1 1 1 1 1 1 1 1 1 1 1 1 1 1]),'partialnetdata',struct('switchedon',0,'format','STD','idmask',['XXXXX XXXXXXXX XXXXXXXX XXXXXXXX'],'idcode','0','idfilter','0','datamaskused',0,'datalength','0','datamask','0x0000000000000000','partialnetworkenable',0)),'blk',['hcu_main_ADASwEPS/RTICANMM' char(10) 'ControllerSetup1'],'allgeneratedfiles',{{'D:\HAITEC\SVN\trunk\ADAS_Softwares\HTDragon\software\sw_development\build\RTICANMM_FILES_ADASwEPS\RTICANMM_SETUP_CAN_2.c','D:\HAITEC\SVN\trunk\ADAS_Softwares\HTDragon\software\sw_development\build\RTICANMM_FILES_ADASwEPS\RTICANMM_SETUP_CAN_2.h','d:\haitec\svn\trunk\adas_softwares\htdragon\software\sw_development\build\rticanmm_files_adasweps\rticanmm_setup_can_2.mexw32'}},'ismp',logical(0),'BlockDataVersion','0.8.0','recreate',0,'CANnedyTag','CAN_2'),'CANnedynew',0,'CANnedySettings','CAN_2','GeneratedFiles',{{'D:\HAITEC\SVN\trunk\ADAS_Softwares\HTDragon\software\sw_development\build\RTICANMM_FILES_ADASwEPS\RTICANMM_SETUP_CAN_2.c','D:\HAITEC\SVN\trunk\ADAS_Softwares\HTDragon\software\sw_development\build\RTICANMM_FILES_ADASwEPS\RTICANMM_SETUP_CAN_2.h','d:\haitec\svn\trunk\adas_softwares\htdragon\software\sw_development\build\rticanmm_files_adasweps\rticanmm_setup_can_2.mexw32'}},'SFCN','RTICANMM_SETUP_CAN_2.c','HostService',struct('Tags',struct('DATA','RTICANMM_MonitorData','TimeStampGlobal','RTICANMM_MonitoringTimeStamp','TimeStampGlobalEnable','RTICANMM_MonitoringTimeStampEnable','Enable','CANMMMonitor_CAN_2','TimeStamp','MonitoringTimeStamp_CAN_2'),'DATA',struct('Length',18),'Info',struct('Desc',{'ID','Service','Data1','Data2','Data3','Data4','Data5','Data6','Data7','Data8','Data9','Data10','Data11','Data12','Data13','Data14','Data15','Data16'}),'Names',struct('TimeStampGlobal','TimeStamp','TimeStampGlobalEnable','TimeStamp_Enable','Enable','Monitoring_Enable','TimeStamp','Monitoring_TimeStamp'),'ChannelID',1)), CANMMType=CANnedySetup, CANMMFolder=D:\HAITEC\SVN\trunk\ADAS_Softwares\HTDragon\software\sw_development\arch, CANMMDestFolder=..\build\RTICANMM_FILES_ADASwEPS, CANMMSettings=CAN_2, CANMMSFcn=RTICANMM_SETUP_CAN_2, CANMMBoard=DS1401, CANMMBoardNum=1, CANMMChannel=2}
      settings: AttributesFormatString=%<CANMMSettings>: %<CANMMBoard>_B%<CANMMBoardNum>_C%<CANMMChannel>  CopyFcn=rticanmm_blockfcn('CopyFcn', 'CANnedySetup', gcb)  DeleteFcn=rticanmm_blockfcn('DeleteFcn', 'CANnedySetup', gcb)  ModelCloseFcn=rticanmm_blockfcn('ModelCloseFcn', 'CANnedySetup', gcb)  NameChangeFcn=rticanmm_blockfcn('NameChangeFcn', 'CANnedySetup', gcb)  OpenFcn=try, rticanmm_setup_gui('create',gcb); ; catch,errordlg({lasterr, '','Please check your RTI installation.'},['Error: ' upper(bdroot)], 'replace'); end  MoveFcn=rticanmm_blockfcn('MoveFcn', 'CANnedySetup', gcb)
      mask Help: eval('rticanmm_quickstart(''create'', gcb);', 'disp(lasterr);')
      mask Display:
      | disp('RTI CAN\nMultiMessage\nControllerSetup')
      | 
      | port_label('input', 1 , 'Variation')
      | port_label('input', 2 , 'Reset')
  RTICANMM GeneralSetup : Subsystem  InitFcn=rticanmm_initfcn(gcb, 'CANnedySettings')  ClipboardFcn=rticanmm_blockfcn('ClipboardFcn', 'CANnedySettings', gcb)  mask(RTICANMM){DSProperties=struct('RTI',struct('Version',uint32(1),'BlockType',struct('isSLSource',uint8(1),'isSLSink',uint8(1),'isHWSource',uint8(0),'isHWSink',uint8(0),'isSetup',uint8(0),'isInline',uint8(1),'isNonInline',uint8(0),'isInterrupt',uint8(0),'isChannelwise',uint8(0)),'IOBoardType','RTICANMM','UnitType','RTICANMM','Identifier','GENERALSETUP','DialogType','SL','BlockSet','RTICANMM','SlaveProcessor','CAN')), CANMMDestFolder=..\build\RTICANMM_FILES_ADASwEPS, CANMMBuildDir=., CANMMAddPaths=on, CANMMAddpathUserMake=on, CANMMRemovePathOnclose=on, CANMMType=CANnedySettings, CANMMProperties=struct('modelroot','D:\HAITEC\SVN\trunk\ADAS_Softwares\HTDragon\software\sw_development\arch','generalsettings',struct('filesettings',struct('destfolder',struct('Name','..\build\RTICANMM_FILES_ADASwEPS','Check',1),'buildfolder',struct('Name','.','Check',1),'AbsDestfolder',struct('Name','D:\HAITEC\SVN\trunk\ADAS_Softwares\HTDragon\software\sw_development\build\RTICANMM_FILES_ADASwEPS'),'AbsBuildfolder',struct('Name','D:\HAITEC\SVN\trunk\ADAS_Softwares\HTDragon\software\sw_development\arch'))),'options',struct('addpaths',1,'rmpaths',1,'addtrcexclusion',1,'cannavigator',struct('checkmonitoring',1),'show_usrtrc',0,'use_usrtrc',0,'addpath2usrmk',1),'advanced',struct('options',[1 1 1 1 1 1 1 1 1 1 1 1 1 1 1 1 1 1 1 1 1 1 1 1 1 1 1 1 1 1 1 1 1 1 1 1 1 1 1 1 1 1 1 1 1 1 1 1 1 1 1 1 1 1 1 1 1 1 1 1 1 1 1 1 1 1 1 1 1 1 1 1 1 1 1 1 1 1 1 1 1 1 1 1 1 1 1 1 1 1 1 1 1 1 1 1 1 1 1 1]),'MPSetup',{{}},'modelname','hcu_main_ADASwEPS','blockdata',struct('generalsettings',struct('filesettings',struct('destfolder',struct('Name','.','Check',1),'AbsDestfolder',struct('Name','T:\TOOL_SOURCES\CANnedy\m'),'buildfolder',struct('Name','.','Check',1),'AbsBuildfolder',struct('Name','C:\MATLAB6p5\work'))),'options',struct('addpaths',1,'rmpaths',1,'addpath2usrmk',1),'modelname','rticanmmlib','modelroot','T:\TOOL_SOURCES\CANnedy\m'),'MMType','RTICANMM','block',['hcu_main_ADASwEPS/RTICANMM' char(10) 'GeneralSetup'],'userdata',struct('HostServiceChannelID',{{'CAN_2',[],'CAN_1'}}),'RTI',struct('Type','RTI1401','Ver','7.4','Date','02-May-2015'),'version','4.1.736021.4900694444')}
      mask prompts: CANMMDestFolder "Destination Folder for generated Files:"; CANMMBuildDir "Build Directory (*_usr.mk, *_usr.trc)"; CANMMAddPaths "Add Paths automatically"; CANMMAddpathUserMake "Add Paths to UserMake-File"; CANMMRemovePathOnclose "Remove added Path on ModelClose"
      mask init:
      | rticanmm_initfcn(gcb,'CANnedyGeneralSettings')
      settings: CopyFcn=rticanmm_blockfcn('CopyFcn', 'CANnedySettings', gcb)  DeleteFcn=rticanmm_blockfcn('DeleteFcn', 'CANnedySettings', gcb)  ModelCloseFcn=rticanmm_blockfcn('CloseFcn', 'CANnedyGeneralSettings', gcb)  NameChangeFcn=rticanmm_blockfcn('NameChangeFcn', 'CANnedySettings', gcb)  OpenFcn=try, rticanmm_gs_gui('create',gcb), ; catch,errordlg({lasterr, '','Please check your RTI installation.'},['Error: ' upper(bdroot)], 'replace'); end  MoveFcn=rticanmm_blockfcn('MoveFcn', 'CANnedySettings', gcb)
      mask Help: eval('rticanmm_quickstart(''create'', gcb);', 'disp(lasterr);')
      mask Display: disp(sprintf(['RTI CAN\nMultiMessage\nGeneralSetup']))
  Reset@RTICANMM ControllerSetup : Constant  Value=0  OutDataTypeStr=boolean
  Reset@RTICANMM ControllerSetup1 : Constant  Value=0  OutDataTypeStr=boolean
  Scheduler : Stateflow chart  TreatAsAtomicUnit=on
  User2CAN1__ : Subsystem
      mask Display: disp('Mapping\nto RTICANMM')
  User2RTICANMM MainBlock_ : Subsystem
      mask Display: disp('Mapping\nto RTICANMM')
  Variation@RTICANMM ControllerSetup : Constant  OutDataTypeStr=uint8
  Variation@RTICANMM ControllerSetup1 : Constant  OutDataTypeStr=uint8
  dHAL_IN : hal/dHAL_IN
  wires:
  Hw_In/1(Hw_In) -> ISP/1(Hw_In)
  OSP/1(OSP_Out) -> Hw_Out/1(OSP_Out)
  ISP/1(ISP_Out) -> EPSS/1(ISP_Out)
  EPSS/2(BEPSS_outputs) -> OSP/2(BEPSS_outputs)
  EPSS/1(BISP_outputs) -> OSP/1(BISP_outputs)
  Scheduler/1(trig_Hw_In()) -> [trig_Hw_In]
  Scheduler/2(trig_ISP()) -> [trig_ISP]
  Scheduler/3(trig_EPSS()) -> [trig_EPSS]
  Scheduler/4(trig_OSP()) -> [trig_OSP]
  Scheduler/5(trig_Hw_Out()) -> [trig_Hw_Out]
  [trig_Hw_In] -> Hw_In/Trigger
  [trig_ISP] -> ISP/Trigger
  [trig_EPSS] -> EPSS/Trigger
  [trig_OSP] -> OSP/Trigger
  [trig_Hw_Out] -> Hw_Out/Trigger
  Scheduler/6(trig_LIDR()) -> [trig_LIDR]
  Scheduler/10(trig_OUTP()) -> [trig_OUTP]
  [trig_LIDR] -> LIDR/Trigger
  Scheduler/7(trig_HAL()) -> [trig_HAL]
  Scheduler/8(trig_INP()) -> [trig_INP]
  Scheduler/9(trig_APP()) -> [trig_APP]
  [trig_HAL] -> dHAL_IN/Trigger
  [trig_APP] -> APPH/Trigger
  Variation@RTICANMM ControllerSetup/1 -> RTICANMM ControllerSetup/1(VariationInput)
  Reset@RTICANMM ControllerSetup/1 -> RTICANMM ControllerSetup/2(Reset)
  Variation@RTICANMM ControllerSetup1/1 -> RTICANMM ControllerSetup1/1(VariationInput)
  Reset@RTICANMM ControllerSetup1/1 -> RTICANMM ControllerSetup1/2(Reset)
  Constant/1 -> INP/1
  [trig_INP] -> INP/Trigger
  INP/1 -> APPH/2(BINP_outputs)
  LIDR/1 -> APPH/1(BLIDR_outputs)
  APPH/2(BDGI_outputs) -> OUTP/2
  APPH/1(BDINR_outputs) -> OUTP/1
  APPH/4(BDFR_outputs) -> OUTP/4
  APPH/3(BDHP_outputs) -> OUTP/3
  [trig_OUTP] -> OUTP/Trigger
  CAN2/1(RX_Data) -> dHAL_IN/2, LIDR/1
  Scheduler/11(trig_CAN()) -> [trig_CAN]
  User2RTICANMM MainBlock_/1(out) -> CAN2/1(TXData)
  CAN1/1(RX_Data) -> ISP/2(CAN_In), User2RTICANMM MainBlock_/1(CAN1_Rx), dHAL_IN/1
  OSP/2(BOSP_outputs) -> User2CAN1__/1(BOSP_outputs)
  OUTP/1 -> User2CAN1__/2(BOUTP_outputs)
  User2CAN1__/1(out) -> CAN1/1(TXData)
  dHAL_IN/1 -> INP/2

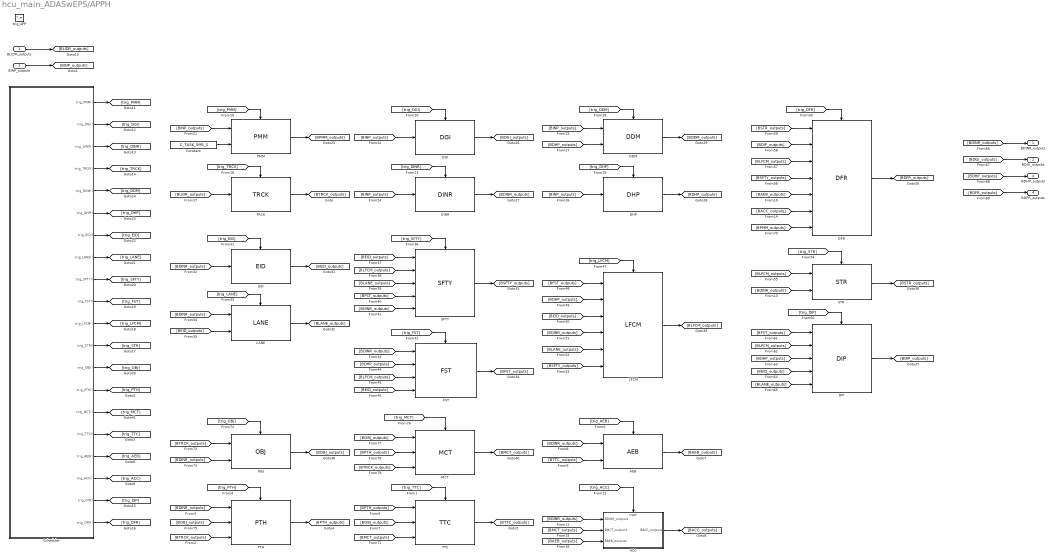
== system hcu_main_ADASwEPS/APPH ==
  BLIDR_outputs : Inport
  BINP_outputs : Inport  Port=2  OutDataTypeStr=Bus: BINP_outputs
      settings: LatchInputForFeedbackSignals=on
  trig_APP : TriggerPort  TriggerType=function-call
  ACC : Subsystem
      settings: RTWSystemCode=Nonreusable function  RTWFcnNameOpts=Use subsystem name  RTWFileNameOpts=Use subsystem name
  AEB : aeb/AEB
  Constant : Constant  Value=C_TASK_5MS_S
  DDM : ddm/DDM
  DFR : dfr/DFR
  DGI : dgi/DGI
  DHP : dhp/DHP
  DINR : dinr/DINR
  DIP : dip/DIP
  EID : eid/EID
  FST : fst/FST
  LANE : lane/LANE
  LFCM : lfcm/LFCM
  MCT : mct/MCT
  OBJ : obj/OBJ
  PMM : pmm/PMM
  PTH : pth/PTH
  SFTY : sfty/SFTY
  STR : str/STR
  Scheduler : Stateflow chart  TreatAsAtomicUnit=on
  TRCK : trck/TRCK
  TTC : ttc/TTC
  BDINR_outputs : Outport  OutDataTypeStr=Bus: BDINR_outputs
  BDGI_outputs : Outport  Port=2  OutDataTypeStr=Bus: BDGI_outputs
  BDHP_outputs : Outport  Port=3  OutDataTypeStr=Bus: BDHP_outputs
  BDFR_outputs : Outport  Port=4  OutDataTypeStr=Bus: BDFR_outputs
  wires:
  BINP_outputs/1 -> [BINP_outputs]
  Scheduler/14(trig_PTH()) -> [trig_PTH]
  [BDINR_outputs] -> PTH/1
  [trig_PTH] -> PTH/Trigger
  PTH/1 -> [BPTH_outputs]
  Scheduler/16(trig_TTC()) -> [trig_TTC]
  [trig_TTC] -> TTC/Trigger
  [BPTH_outputs] -> TTC/1
  [BOBJ_outputs] -> TTC/2
  TTC/1 -> [BTTC_outputs]
  Scheduler/17(trig_AEB()) -> [trig_AEB]
  [trig_AEB] -> AEB/Trigger
  [BDINR_outputs] -> AEB/1
  [BTTC_outputs] -> AEB/2
  AEB/1 -> [BAEB_outputs]
  ACC/1(BACC_outputs) -> [BACC_outputs]
  [trig_ACC] -> ACC/Trigger
  Scheduler/18(trig_ACC()) -> [trig_ACC]
  [BMCT_outputs] -> ACC/2(BMCT_outputs)
  TRCK/1 -> [BTRCK_outputs]
  BLIDR_outputs/1 -> [BLIDR_outputs]
  [BLIDR_outputs] -> TRCK/1
  Scheduler/1(trig_PMM()) -> [trig_PMM]
  Scheduler/2(trig_DGI()) -> [trig_DGI]
  Scheduler/3(trig_DINR()) -> [trig_DINR]
  Scheduler/4(trig_TRCK()) -> [trig_TRCK]
  [trig_TRCK] -> TRCK/Trigger
  Scheduler/19(trig_DIP()) -> [trig_DIP]
  Scheduler/20(trig_DFR()) -> [trig_DFR]
  Scheduler/12(trig_STR()) -> [trig_STR]
  Scheduler/11(trig_LFCM()) -> [trig_LFCM]
  Scheduler/10(trig_FST()) -> [trig_FST]
  Scheduler/9(trig_SFTY()) -> [trig_SFTY]
  Scheduler/8(trig_LANE()) -> [trig_LANE]
  Scheduler/7(trig_EID()) -> [trig_EID]
  Scheduler/6(trig_DHP()) -> [trig_DHP]
  Scheduler/5(trig_DDM()) -> [trig_DDM]
  [trig_PMM] -> PMM/Trigger
  [BINP_outputs] -> PMM/1
  Constant/1 -> PMM/2
  PMM/1 -> [BPMM_outputs]
  [trig_DGI] -> DGI/Trigger
  [BINP_outputs] -> DGI/1
  DGI/1 -> [BDGI_outputs]
  [trig_DINR] -> DINR/Trigger
  [BINP_outputs] -> DINR/1
  DINR/1 -> [BDINR_outputs]
  [BINP_outputs] -> DDM/1
  [BINP_outputs] -> DHP/1
  [BDHP_outputs] -> DDM/2
  DHP/1 -> [BDHP_outputs]
  DDM/1 -> [BDDM_outputs]
  [trig_DDM] -> DDM/Trigger
  [trig_DHP] -> DHP/Trigger
  [trig_DFR] -> DFR/Trigger
  DFR/1 -> [BDFR_outputs]
  [trig_EID] -> EID/Trigger
  [BDINR_outputs] -> EID/1
  EID/1 -> [BEID_outputs]
  [trig_LANE] -> LANE/Trigger
  [BDINR_outputs] -> LANE/1
  [BEID_outputs] -> LANE/2
  LANE/1 -> [BLANE_outputs]
  [trig_SFTY] -> SFTY/Trigger
  [BEID_outputs] -> SFTY/1
  [BLFCM_outputs] -> SFTY/2
  [BLANE_outputs] -> SFTY/3
  [BFST_outputs] -> SFTY/4
  [BDINR_outputs] -> SFTY/5
  [trig_FST] -> FST/Trigger
  [BDINR_outputs] -> FST/1
  [BDHP_outputs] -> FST/2
  [BLFCM_outputs] -> FST/3
  [BEID_outputs] -> FST/4
  SFTY/1 -> [BSFTY_outputs]
  FST/1 -> [BFST_outputs]
  [trig_LFCM] -> LFCM/Trigger
  [BFST_outputs] -> LFCM/1
  [BDHP_outputs] -> LFCM/2
  [BEID_outputs] -> LFCM/3
  [BDINR_outputs] -> LFCM/4
  [BLANE_outputs] -> LFCM/5
  [BSFTY_outputs] -> LFCM/6
  LFCM/1 -> [BLFCM_outputs]
  [trig_STR] -> STR/Trigger
  [BLFCM_outputs] -> STR/1
  STR/1 -> [BSTR_outputs]
  [BSFTY_outputs] -> DFR/4
  [BLFCM_outputs] -> DFR/3
  [BDIP_outputs] -> DFR/2
  [BSTR_outputs] -> DFR/1
  [trig_DIP] -> DIP/Trigger
  [BFST_outputs] -> DIP/1
  [BLFCM_outputs] -> DIP/2
  [BDHP_outputs] -> DIP/3
  [BEID_outputs] -> DIP/4
  [BLANE_outputs] -> DIP/5
  DIP/1 -> [BDIP_outputs]
  [BDINR_outputs] -> BDINR_outputs/1
  [BDGI_outputs] -> BDGI_outputs/1
  [BDHP_outputs] -> BDHP_outputs/1
  [BDFR_outputs] -> BDFR_outputs/1
  [BDINR_outputs] -> ACC/1(BDINR_outputs)
  [BAEB_outputs] -> DFR/5
  [BACC_outputs] -> DFR/6
  [BPMM_outputs] -> DFR/7
  [BMCT_outputs] -> TTC/3
  [BTRCK_outputs] -> OBJ/1
  [BDINR_outputs] -> OBJ/2
  OBJ/1 -> [BOBJ_outputs]
  [trig_OBJ] -> OBJ/Trigger
  Scheduler/13(trig_OBJ()) -> [trig_OBJ]
  [BTRCK_outputs] -> PTH/3
  [BOBJ_outputs] -> PTH/2
  [trig_MCT] -> MCT/Trigger
  MCT/1 -> [BMCT_outputs]
  [BOBJ_outputs] -> MCT/1
  [BPTH_outputs] -> MCT/2
  [BTRCK_outputs] -> MCT/3
  Scheduler/15(trig_MCT()) -> [trig_MCT]
  [BDINR_outputs] -> STR/2
  [BAEB_outputs] -> ACC/3(BAEB_outputs)
